simulink model "aquaMasterModel"  (R2023b)
settings: Solver=VariableStepAuto  StartTime=0.0  StopTime=Tfinal  FixedStep=dt_sc  MaxStep=0.25  RelTol=1e-3
model workspace (MAT data in the model file):
  R0 = [-0.985692836836  -0.0898143567564  0.142628933706; 0.00615410867898  -0.864816584843  -0.502050198215; 0.168439182959  -0.493989530154  0.852996240169]
  R_des = [0  0  -1; 0  1  0; 1  0  0]
  Tfinal = 30
  om0 = [0.0019806286476; 0.00760530712199; 0.176224033565]
  om_des = [-0.00105965330436; 0; 0]
  targetAttitude.R_des = timeseries
  targetAttitude.R_des.Name = 'unnamed'
  targetAttitude.R_des.DataInfo = tsdata.datametadata
  targetAttitude.R_des.DataInfo.Interpolation = tsdata.interpolation
  targetAttitude.R_des.DataInfo.Interpolation.Fhandle : function handle (value not decoded)
  targetAttitude.R_des.DataInfo.Interpolation.Name = 'linear'
  targetAttitude.R_des.TimeInfo = tsdata.timemetadata
  targetAttitude.R_des.TimeInfo.Length = 2
  targetAttitude.R_des.TimeInfo.DuplicateTimes = 0
  targetAttitude.R_des.TimeInfo.Time_ = [0; 17788.4180081]
  targetAttitude.R_des.TimeInfo.Initialized = 1
  targetAttitude.R_des.QualityInfo = tsdata.qualmetadata
  targetAttitude.R_des.Data_ = reshape([-0.985692836836 0.00615410867898 0.168439182959 -0.0898143567564 -0.864816584843 -0.493989530154 0.142628933706 -0.502050198215 0.852996240169 -0.985692836836 0.00615410867898 0.168439182959 -0.0898143567564 -0.864816584843 -0.493989530154 0.142628933706 -0.502050198215 0.852996240169], [3 3 2])
  targetAttitude.om_des = timeseries
  targetAttitude.om_des.Name = 'unnamed'
  targetAttitude.om_des.DataInfo = tsdata.datametadata
  targetAttitude.om_des.DataInfo.Interpolation = tsdata.interpolation
  targetAttitude.om_des.DataInfo.Interpolation.Fhandle : function handle (value not decoded)
  targetAttitude.om_des.DataInfo.Interpolation.Name = 'linear'
  targetAttitude.om_des.TimeInfo = tsdata.timemetadata
  targetAttitude.om_des.TimeInfo.Length = 2
  targetAttitude.om_des.TimeInfo.DuplicateTimes = 0
  targetAttitude.om_des.TimeInfo.Time_ = [0; 17788.4180081]
  targetAttitude.om_des.TimeInfo.Initialized = 1
  targetAttitude.om_des.QualityInfo = tsdata.qualmetadata
  targetAttitude.om_des.Data_ = reshape([0 -0.00105965330436 0 0 -0.00105965330436 0], [3 1 2])
  u0 = [0.00088339814174; 0.00685359918368; 0.00953393346195]
values from neighbouring files (symbols this model uses):
  A_ptob = [0.00452111179393  0.994865050863  -0.101109297888; -0.99864921572  -0.000741813086313  -0.051953764597; -0.0517619888586  0.101207609816  0.993517848971]    [magConstants.mat]
undefined symbols (not defined in the file or in its folder): Itotal_p
libraries: rotationConversionLib x2, matrix_library x1
settings Model: PacingRate=50  Creator=kristopherriordan  LastModifiedBy=kristopherriordan
settings ModelReferenceCC: ModelReferenceMinAlgLoopOccurrences=on

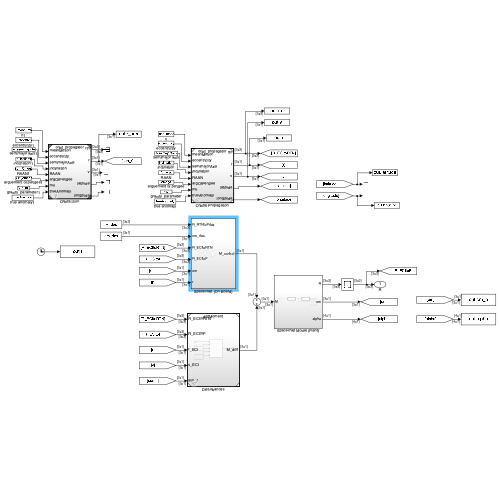
[thumbnail: Simulink's stored preview of the top-level diagram]
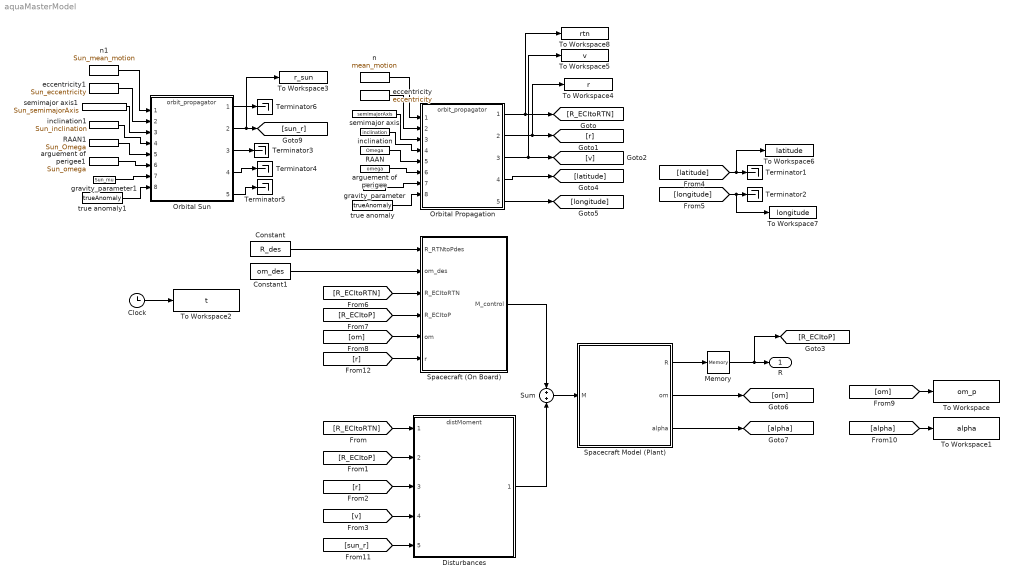
== system aquaMasterModel ==
  Clock : Clock
  Constant : Constant  Value=R_des  VectorParams1D=off
  Constant1 : Constant  Value=om_des  VectorParams1D=off
  Disturbances : ModelReference  ModelNameDialog=distMoment.slx  SimulationMode=Normal  ModelReferenceVersion=1.196
  Memory : Memory  InitialCondition=R0  InheritSampleTime=on
  Orbital Propagation : ModelReference  ModelNameDialog=orbit_propagator.slx  SimulationMode=Normal  ModelReferenceVersion=1.31
  Orbital Sun : ModelReference  ModelNameDialog=orbit_propagator.slx  SimulationMode=Normal  ModelReferenceVersion=1.31
  RAAN : FromWorkspace  VariableName=Omega
  RAAN1 : FromWorkspace  VariableName=Sun_Omega
  Spacecraft (On Board) : Subsystem
  Spacecraft Model (Plant) : Subsystem
  Sum : Sum  Inputs=+|+
  Terminator{1..6} (6 alike) : Terminator
  To Workspace : ToWorkspace  VariableName=om_p  SaveFormat=Timeseries  SampleTime=-1
  To Workspace1 : ToWorkspace  VariableName=alpha  SaveFormat=Timeseries  SampleTime=-1
  To Workspace2 : ToWorkspace  VariableName=t  SampleTime=-1
      settings: Save2DSignal=2-D array (concatenate along first dimension)
  To Workspace3 : ToWorkspace  VariableName=r_sun  SaveFormat=Timeseries  SampleTime=-1
  To Workspace4 : ToWorkspace  VariableName=r  SaveFormat=Timeseries  SampleTime=-1
  To Workspace5 : ToWorkspace  VariableName=v  SaveFormat=Timeseries  SampleTime=-1
  To Workspace6 : ToWorkspace  VariableName=latitude  SaveFormat=Timeseries  SampleTime=-1
  To Workspace7 : ToWorkspace  VariableName=longitude  SaveFormat=Timeseries  SampleTime=-1
  To Workspace8 : ToWorkspace  VariableName=rtn  SaveFormat=Timeseries  SampleTime=-1
  arguement of perigee : FromWorkspace  VariableName=omega
  arguement of perigee1 : FromWorkspace  VariableName=Sun_omega
  eccentricity : FromWorkspace  VariableName=eccentricity
  eccentricity1 : FromWorkspace  VariableName=Sun_eccentricity
  gravity_parameter : FromWorkspace  VariableName=mu
  gravity_parameter1 : FromWorkspace  VariableName=Sun_mu
  inclination : FromWorkspace  VariableName=inclination
  inclination1 : FromWorkspace  VariableName=Sun_inclination
  n : FromWorkspace  VariableName=mean_motion
  n1 : FromWorkspace  VariableName=Sun_mean_motion
  semimajor axis : FromWorkspace  VariableName=semimajorAxis  OutDataTypeStr=double
  semimajor axis1 : FromWorkspace  VariableName=Sun_semimajorAxis  OutDataTypeStr=double
  true anomaly : FromWorkspace  VariableName=trueAnomaly
  true anomaly1 : FromWorkspace  VariableName=trueAnomaly
  R : Outport
  wires:
  Disturbances/1 -> Sum/2
  [R_ECItoRTN] -> Disturbances/1
  [R_ECItoP] -> Disturbances/2
  [r] -> Disturbances/3
  [v] -> Disturbances/4
  Memory/1 -> R/1, [R_ECItoP]
  Orbital Propagation/5 -> [longitude]
  Orbital Propagation/4 -> [latitude]
  Spacecraft Model (Plant)/1(R) -> Memory/1
  Spacecraft Model (Plant)/2(om) -> [om]
  [R_ECItoRTN] -> Spacecraft (On Board)/3(R_ECItoRTN)
  [R_ECItoP] -> Spacecraft (On Board)/4(R_ECItoP)
  [om] -> Spacecraft (On Board)/5(om)
  Spacecraft (On Board)/1(M_control) -> Sum/1
  Spacecraft Model (Plant)/3(alpha) -> [alpha]
  [om] -> To Workspace/1
  [alpha] -> To Workspace1/1
  Clock/1 -> To Workspace2/1
  n/1 -> Orbital Propagation/1
  eccentricity/1 -> Orbital Propagation/2
  semimajor axis/1 -> Orbital Propagation/3
  inclination/1 -> Orbital Propagation/4
  RAAN/1 -> Orbital Propagation/5
  arguement of perigee/1 -> Orbital Propagation/6
  gravity_parameter/1 -> Orbital Propagation/7
  true anomaly/1 -> Orbital Propagation/8
  Orbital Sun/3 -> Terminator3/1
  n1/1 -> Orbital Sun/1
  true anomaly1/1 -> Orbital Sun/8
  Orbital Sun/5 -> Terminator5/1
  Orbital Sun/4 -> Terminator4/1
  arguement of perigee1/1 -> Orbital Sun/6
  Orbital Sun/1 -> Terminator6/1
  semimajor axis1/1 -> Orbital Sun/3
  gravity_parameter1/1 -> Orbital Sun/7
  RAAN1/1 -> Orbital Sun/5
  eccentricity1/1 -> Orbital Sun/2
  inclination1/1 -> Orbital Sun/4
  Orbital Sun/2 -> To Workspace3/1, [sun_r]
  Orbital Propagation/2 -> To Workspace4/1, [r]
  Orbital Propagation/3 -> To Workspace5/1, [v]
  [latitude] -> To Workspace6/1, Terminator1/1
  [longitude] -> To Workspace7/1, Terminator2/1
  Orbital Propagation/1 -> To Workspace8/1, [R_ECItoRTN]
  [sun_r] -> Disturbances/5
  [r] -> Spacecraft (On Board)/6(r)
  Sum/1 -> Spacecraft Model (Plant)/1(M)
  Constant/1 -> Spacecraft (On Board)/1(R_RTNtoPdes)
  Constant1/1 -> Spacecraft (On Board)/2(om_des)

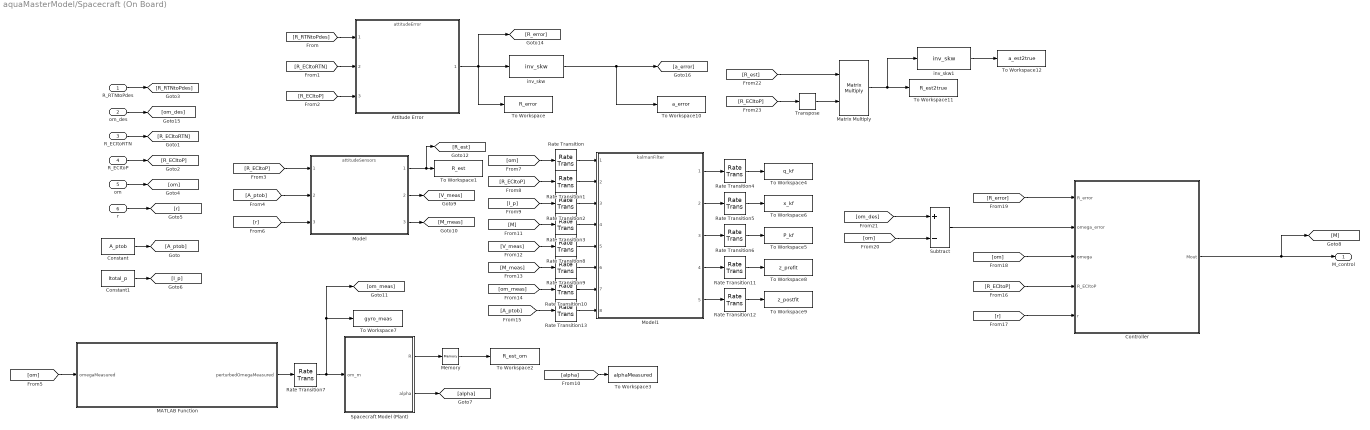
== system aquaMasterModel/Spacecraft (On Board) ==
  R_RTNtoPdes : Inport
  om_des : Inport  Port=2
  R_ECItoRTN : Inport  Port=3
  R_ECItoP : Inport  Port=4
  om : Inport  Port=5
  r : Inport  Port=6
  Attitude Error : ModelReference  ModelNameDialog=attitudeError.slx  SimulationMode=Normal  ModelReferenceVersion=1.7
  Constant : Constant  Value=A_ptob  VectorParams1D=off
  Constant1 : Constant  Value=Itotal_p  VectorParams1D=off
  Controller : Subsystem
  MATLAB Function : MATLAB Function  TreatAsAtomicUnit=on
  Matrix Multiply : Product  Multiplication=Matrix(*)
  Memory : Memory  InitialCondition=R0  InheritSampleTime=on
  Model : ModelReference  ModelNameDialog=attitudeSensors.slx  SimulationMode=Normal  ModelReferenceVersion=1.107
  Model1 : ModelReference  ModelNameDialog=kalmanFilter.slx  SimulationMode=Normal  ModelReferenceVersion=1.248
  Rate Transition{,1..13} (14 alike) : RateTransition
  Spacecraft Model (Plant) : Subsystem
  Subtract : Sum  Inputs=+-
  To Workspace : ToWorkspace  VariableName=R_error  SaveFormat=Timeseries  SampleTime=-1
  To Workspace1 : ToWorkspace  VariableName=R_est  SaveFormat=Timeseries  SampleTime=-1
  To Workspace10 : ToWorkspace  VariableName=a_error  SaveFormat=Timeseries  SampleTime=-1
  To Workspace11 : ToWorkspace  VariableName=R_est2true  SaveFormat=Timeseries  SampleTime=-1
  To Workspace12 : ToWorkspace  VariableName=a_est2true  SaveFormat=Timeseries  SampleTime=-1
  To Workspace2 : ToWorkspace  VariableName=R_est_om  SaveFormat=Timeseries  SampleTime=-1
  To Workspace3 : ToWorkspace  VariableName=alphaMeasured  SaveFormat=Timeseries  SampleTime=-1
  To Workspace4 : ToWorkspace  VariableName=q_kf  SaveFormat=Timeseries  SampleTime=-1
  To Workspace5 : ToWorkspace  VariableName=P_kf  SaveFormat=Timeseries  SampleTime=-1
  To Workspace6 : ToWorkspace  VariableName=x_kf  SaveFormat=Timeseries  SampleTime=-1
  To Workspace7 : ToWorkspace  VariableName=gyro_meas  SaveFormat=Timeseries  SampleTime=-1
  To Workspace8 : ToWorkspace  VariableName=z_prefit  SaveFormat=Timeseries  SampleTime=-1
  To Workspace9 : ToWorkspace  VariableName=z_postfit  SaveFormat=Timeseries  SampleTime=-1
  Transpose : matrix_library/Transpose
  inv_skw : rotationConversionLib/inv_skw  SystemSampleTime=-1  VariantActivationTime=update diagram  AllowFlexibleInterface=on  Latency=0  AutoFrameSizeCalculation=off
  inv_skw1 : rotationConversionLib/inv_skw  SystemSampleTime=-1  VariantActivationTime=update diagram  AllowFlexibleInterface=on  Latency=0  AutoFrameSizeCalculation=off
  M_control : Outport
  wires:
  R_RTNtoPdes/1 -> [R_RTNtoPdes]
  R_ECItoRTN/1 -> [R_ECItoRTN]
  R_ECItoP/1 -> [R_ECItoP]
  om/1 -> [om]
  [R_RTNtoPdes] -> Attitude Error/1
  Attitude Error/1 -> inv_skw/1, [R_error], To Workspace/1
  Model/1 -> [R_est], To Workspace1/1
  [R_ECItoP] -> Model/1
  Constant/1 -> [A_ptob]
  [A_ptob] -> Model/2
  Memory/1 -> To Workspace2/1
  Spacecraft Model (Plant)/1(R) -> Memory/1
  [alpha] -> To Workspace3/1
  Spacecraft Model (Plant)/2(alpha) -> [alpha]
  r/1 -> [r]
  [r] -> Model/3
  [om] -> MATLAB Function/1(omegaMeasured)
  [om] -> Rate Transition/1
  [R_ECItoP] -> Rate Transition1/1
  [I_p] -> Rate Transition2/1
  Constant1/1 -> [I_p]
  [M] -> Rate Transition3/1
  Rate Transition/1 -> Model1/1
  Rate Transition1/1 -> Model1/2
  Rate Transition2/1 -> Model1/3
  Rate Transition3/1 -> Model1/4
  Model1/2 -> Rate Transition5/1
  Model1/3 -> Rate Transition6/1
  Model1/1 -> Rate Transition4/1
  Rate Transition4/1 -> To Workspace4/1
  Rate Transition5/1 -> To Workspace6/1
  Rate Transition6/1 -> To Workspace5/1
  MATLAB Function/1(perturbedOmegaMeasured) -> Rate Transition7/1
  Rate Transition7/1 -> Spacecraft Model (Plant)/1(om_m), [om_meas], To Workspace7/1
  [V_meas] -> Rate Transition8/1
  [M_meas] -> Rate Transition9/1
  [om_meas] -> Rate Transition10/1
  Rate Transition8/1 -> Model1/5
  Rate Transition9/1 -> Model1/6
  Rate Transition10/1 -> Model1/7
  Model/2 -> [V_meas]
  Model/3 -> [M_meas]
  Model1/4 -> Rate Transition11/1
  Model1/5 -> Rate Transition12/1
  Rate Transition11/1 -> To Workspace8/1
  Rate Transition12/1 -> To Workspace9/1
  [A_ptob] -> Rate Transition13/1
  Rate Transition13/1 -> Model1/8
  [r] -> Controller/5(r)
  [R_ECItoP] -> Controller/4(R_ECItoP)
  [om] -> Controller/3(omega)
  [R_error] -> Controller/1(R_error)
  Subtract/1 -> Controller/2(omega_error)
  [om] -> Subtract/2
  [om_des] -> Subtract/1
  om_des/1 -> [om_des]
  inv_skw/1 -> To Workspace10/1, [a_error]
  [R_ECItoRTN] -> Attitude Error/2
  [R_ECItoP] -> Attitude Error/3
  [R_ECItoP] -> Transpose/1
  Transpose/1 -> Matrix Multiply/2
  [R_est] -> Matrix Multiply/1
  Matrix Multiply/1 -> inv_skw1/1, To Workspace11/1
  inv_skw1/1 -> To Workspace12/1
  Controller/1(Mout) -> M_control/1, [M]

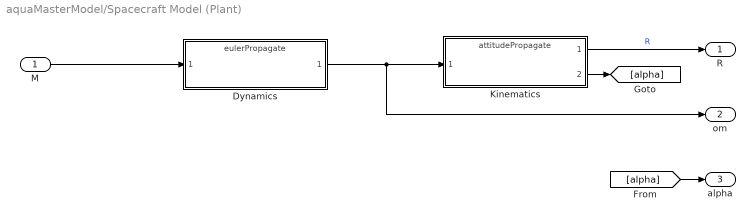
== system aquaMasterModel/Spacecraft Model (Plant) ==
  M : Inport
  Dynamics : ModelReference  ModelNameDialog=eulerPropagate.slx  SimulationMode=Normal  ModelReferenceVersion=1.38
  Kinematics : ModelReference  ModelNameDialog=attitudePropagate.slx  SimulationMode=Normal  ModelReferenceVersion=1.208
  R : Outport
  om : Outport  Port=2
  alpha : Outport  Port=3
  wires:
  Kinematics/1 -> R/1  "R"
  Dynamics/1 -> om/1, Kinematics/1
  M/1 -> Dynamics/1
  Kinematics/2 -> [alpha]
  [alpha] -> alpha/1

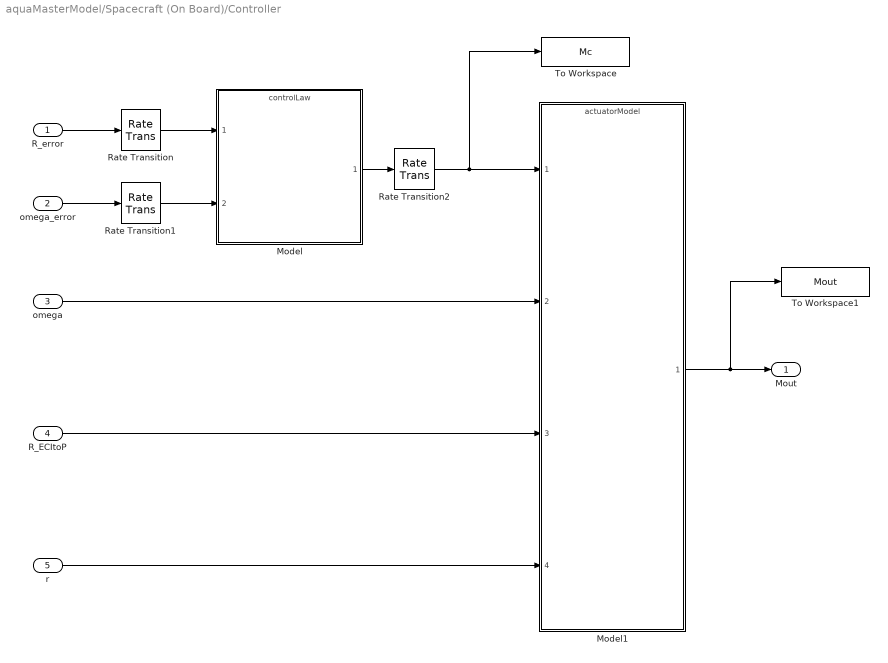
== system aquaMasterModel/Spacecraft (On Board)/Controller ==
  R_error : Inport
  omega_error : Inport  Port=2
  omega : Inport  Port=3
  R_ECItoP : Inport  Port=4
  r : Inport  Port=5
  Model : ModelReference  ModelNameDialog=controlLaw.slx  SimulationMode=Normal  ModelReferenceVersion=1.89
  Model1 : ModelReference  ModelNameDialog=actuatorModel.slx  SimulationMode=Normal  ModelReferenceVersion=1.98
  Rate Transition : RateTransition
  Rate Transition1 : RateTransition
  Rate Transition2 : RateTransition
  To Workspace : ToWorkspace  VariableName=Mc  SaveFormat=Timeseries  SampleTime=-1
  To Workspace1 : ToWorkspace  VariableName=Mout  SaveFormat=Timeseries  SampleTime=-1
  Mout : Outport
  wires:
  Model1/1 -> To Workspace1/1, Mout/1
  omega/1 -> Model1/2
  Model/1 -> Rate Transition2/1
  omega_error/1 -> Rate Transition1/1
  R_error/1 -> Rate Transition/1
  R_ECItoP/1 -> Model1/3
  r/1 -> Model1/4
  Rate Transition/1 -> Model/1
  Rate Transition1/1 -> Model/2
  Rate Transition2/1 -> To Workspace/1, Model1/1

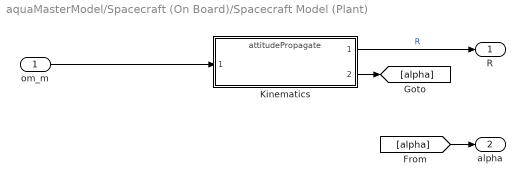
== system aquaMasterModel/Spacecraft (On Board)/Spacecraft Model (Plant) ==
  om_m : Inport
  Kinematics : ModelReference  ModelNameDialog=attitudePropagate.slx  SimulationMode=Normal  ModelReferenceVersion=1.208
  R : Outport
  alpha : Outport  Port=2
  wires:
  Kinematics/1 -> R/1  "R"
  om_m/1 -> Kinematics/1
  Kinematics/2 -> [alpha]
  [alpha] -> alpha/1

== matlab function aquaMasterModel/Spacecraft (On Board)/MATLAB Function ==
  settings: updateMethod=DISCRETE  sampleTime=dt_sc
  data: omegaMeasured input; perturbedOmegaMeasured output
function perturbedOmegaMeasured = OmegaMeasurementErrors(omegaMeasured)

% Convert degrees per second to radians per second for bias error
bias_error_deg_per_sec = 0.00; % Example bias error in degrees per second (from Bosch BMI160)
bias_error_rad_per_sec = bias_error_deg_per_sec * (pi / 180); % Convert to radians per second

% Convert noise density to standard deviation for a given bandwidth
noise_density_deg_per_sec_sqrtHz = 0.014; % Example noise density in degrees per second per sqrt(Hz)
% noise_density_deg_per_sec_sqrtHz = 0;
bandwidth = 1; % Assuming a bandwidth of 1 Hz for simplicity
noise_std_dev_deg_per_sec = noise_density_deg_per_sec_sqrtHz * sqrt(bandwidth); % Standard deviation in degrees per second
noise_std_dev_rad_per_sec = noise_std_dev_deg_per_sec * (pi / 180); % Convert to radians per second

% Bias error (constant offset)
bias_error = bias_error_rad_per_sec .* ones(size(omegaMeasured));

% Generate Gaussian noise
noise = noise_std_dev_rad_per_sec .* randn(size(omegaMeasured));


% Add the errors to the unit vector
error = bias_error + noise;
perturbedOmegaMeasured = error + omegaMeasured;
